simulink model "simulation_pipeline"  (R2023a)
settings: Solver=VariableStepAuto  StartTime=0.0  StopTime=10  FixedStep=1/2000  RelTol=1e-3
model workspace (MAT data in the model file):
  a = Simulink.Parameter
  a.Value = [0.16054 0.65442]
  a.DataType = 'auto'
  a.Complexity = 'real'
  a.Dimensions = [1 2]
  b = Simulink.Parameter
  b.Value = [0.16054 0.65442 1]
  b.DataType = 'auto'
  b.Complexity = 'real'
  b.Dimensions = [1 3]
  c = Simulink.Parameter
  c.Value = [1 1]
  c.DataType = 'auto'
  c.Complexity = 'real'
  c.Dimensions = [1 2]
  g = Simulink.Parameter
  g.Value = 0.00080298
  g.DataType = 'auto'
  g.Complexity = 'real'
  g.Dimensions = [1 1]
undefined symbols (not defined in the file): firhalfband
libraries: dspmlti4 x3, msbAdcFoundation x1, dspsigops x1, dspquant2 x1
settings Model: Creator=Lester  LastModifiedBy=Lester
settings DataIOCC: ReturnWorkspaceOutputs=off

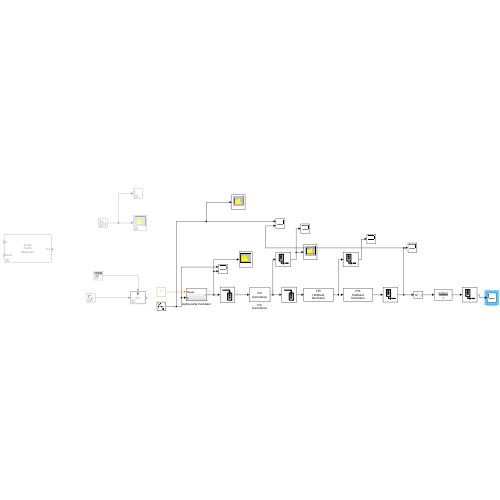
[thumbnail: Simulink's stored preview of the top-level diagram]
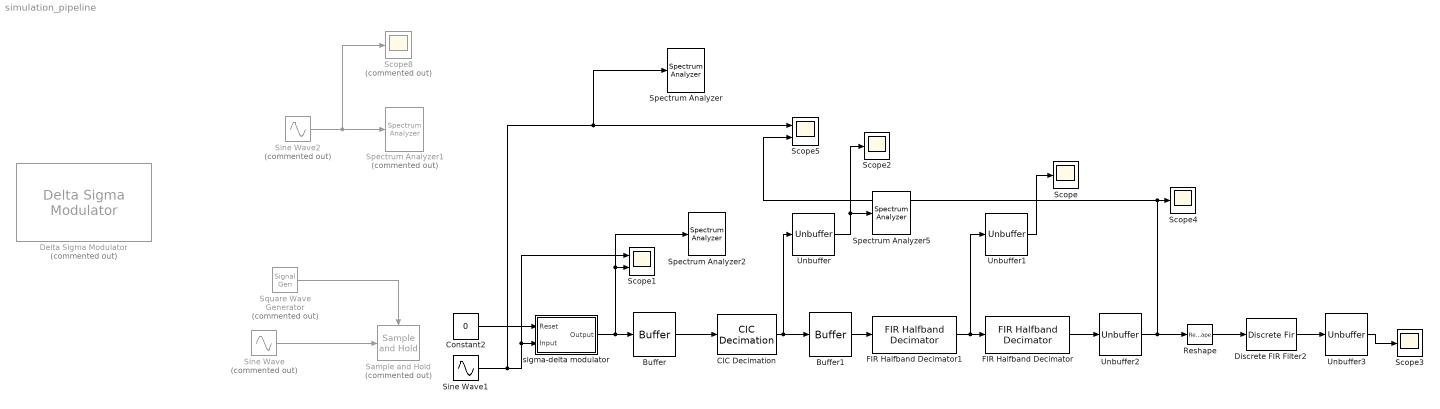
== system simulation_pipeline ==
  Buffer : Buffer  N=24  OutputFrames=off
  Buffer1 : Buffer  N=8  OutputFrames=off
  CIC Decimation : dspmlti4/CIC Decimation  filtFrom=Dialog parameters  filtobj=CICDECIM  ftype=Decimator  R=12  M=1  N=4  filterInternals=Full precision  BPS=[16 16 16 16]  FLPS=0  outputWordLength=32  outputFracLength=0  launchFVT=off  framing=Maintain input frame rate  RateOptions=Enforce single-rate processing
      settings: LibrarySourceBlock=|
      | dsphdlsupportfiltering/CIC
      | Decimation
  Constant2 : Constant  Value=0  SampleTime=1/2.304e6
  Delta Sigma Modulator : msbAdcFoundation/Delta Sigma Modulator  Commented=on  dsmArchitecture=CIFB  dsmOrder=2nd order  SamplingFrequency=128e3  NumberLevels=2  QuantizerOutput=[-1;1]  a=[0.1601 0.6515]  g=[0.0]  b=[0.1601 0.6515 1]  c=[1 1]  EnableNoise=on  SNR=75  InputPower=0.125  BandWidth=1000
      link override Delta Sigma Modulator: LabelModeActiveChoice=2CIFB
      link override Noise: LabelModeActiveChoice=noise
  Discrete FIR Filter2 : DiscreteFir  Coefficients=|  SampleTime=96e3
      | [-0.000958177958379201246547074433124180359
      | -0.003782484366489099070901547250400653866
      | -0.008055996906683227792855817028794263024
      | -0.010365278062492658955884294869065342937
      | -0.00550473485434811379835018385620060144 
      |  0.008631607068306285449055259562101127813
      |  0.025719525280152786411713705660986306611
      |  0.031614424562770325477512045608818880282
      |  0.014320649256157549564227871030652750051
      | -0.022003543765387822972456888237502425909
      | -0.051505493094117581198698729849638766609
      | -0.038973297856755691193075819001023774035
      |  0.034481095551837454005195127137994859368
      |  0.150902569099642724914644986711209639907
      |  0.25888391496113211109886265148816164583 
      |  0.302836379627961560512261485200724564493
      |  0.25888391496113211109886265148816164583 
      |  0.150902569099642724914644986711209639907
      |  0.034481095551837454005195127137994859368
      | -0.038973297856755691193075819001023774035
      | -0.051505493094117581198698729849638766609
      | -0.022003543765387822972456888237502425909
      |  0.014320649256157549564227871030652750051
      |  0.031614424562770325477512045608818880282
      |  0.025719525280152786411713705660986306611
      |  0.008631607068306285449055259562101127813
      | -0.00550473485434811379835018385620060144 
      | -0.010365278062492658955884294869065342937
      | -0.008055996906683227792855817028794263024
      | -0.003782484366489099070901547250400653866
      | -0.000958177958379201246547074433124180359]
  FIR Halfband Decimator : dspmlti4/FIR Halfband Decimator  Specification=Filter order and stopband attenuation  FilterOrder=14  TransitionWidth=4.1e3  StopbandAttenuation=100  DesignMethod=Auto  Numerator=firhalfband( 'minorder', 0.407, 1e-4 )  FilterBankOutputPort=off  InheritSampleRate=off  SampleRate=96e3  SimulateUsing=Code generation  roundingMode=Floor  coeffsDataTypeStr=fixdt(1,16)
  FIR Halfband Decimator1 : dspmlti4/FIR Halfband Decimator  Specification=Filter order and stopband attenuation  FilterOrder=14  TransitionWidth=4.1e3  StopbandAttenuation=100  DesignMethod=Auto  Numerator=firhalfband( 'minorder', 0.407, 1e-4 )  FilterBankOutputPort=off  InheritSampleRate=off  SampleRate=2*96e3  SimulateUsing=Code generation  roundingMode=Floor  coeffsDataTypeStr=fixdt(1,16)
  Reshape : Reshape  OutputDimensions=[1,2]
  Sample and Hold : dspsigops/Sample and Hold  Commented=on  trig=Rising edge  initCond=0  latchinput=off
  Scope{,2..4} (4 alike) : Scope
  Scope1 : Scope  NumInputPorts=2
  Scope5 : Scope  NumInputPorts=2
  Scope8 : Scope  Commented=on
  Sine Wave : Sin  Commented=on  Frequency=2*pi*100  SampleTime=1/2.304e6
  Sine Wave1 : Sin  Frequency=2*pi*100  SampleTime=1/2.304e6
  Sine Wave2 : Sin  Commented=on  Frequency=2*pi*100  SampleTime=1/2000
  Spectrum Analyzer : SpectrumAnalyzer  WindowPosition=[1.000000,49.000000,1707.000000,889.000000,]  ScopeFrameLocation=window  SpectrumType=Power density  SpectrumUnits=dBm/Hz  YLimits=[-308.65856886,26.07461712]  ColorLimits=[-80 20]
  Spectrum Analyzer1 : SpectrumAnalyzer  Commented=on  WindowPosition=[1.000000,49.000000,1707.000000,889.000000,]  ScopeFrameLocation=window  YLimits=[-240.74775427,-25.54872748]  ColorLimits=[-80 20]
  Spectrum Analyzer2 : SpectrumAnalyzer  WindowPosition=[1.000000,49.000000,1707.000000,889.000000,]  ScopeFrameLocation=window  SpectrumType=Power density  SpectrumUnits=dBm/Hz  YLimits=[-107.56343722,4.98269637]  ColorLimits=[-80 20]
  Spectrum Analyzer5 : SpectrumAnalyzer  WindowPosition=[1.000000,49.000000,1707.000000,889.000000,]  ScopeFrameLocation=window  SpectrumType=Power density  SpectrumUnits=dBm/Hz  YLimits=[-25.98451667,95.0310336]  ColorLimits=[-80 20]
  Square Wave Generator : SignalGenerator  Commented=on  WaveForm=square  Frequency=2.304e6  VectorParams1D=off
  Unbuffer{,1..3} (4 alike) : Unbuffer
  sigma-delta modulator : Subsystem
  wires:
  Square Wave Generator/1 -> Sample and Hold/Trigger
  Sine Wave/1 -> Sample and Hold/1
  Constant2/1 -> sigma-delta modulator/1(Reset)
  sigma-delta modulator/1(Output) -> Buffer/1, Spectrum Analyzer2/1, Scope1/2
  CIC Decimation/1 -> Unbuffer/1, Buffer1/1
  FIR Halfband Decimator1/1 -> Unbuffer1/1, FIR Halfband Decimator/1
  FIR Halfband Decimator/1 -> Unbuffer2/1
  Buffer/1 -> CIC Decimation/1
  Sine Wave1/1 -> Spectrum Analyzer/1, Scope5/1, Scope1/1, sigma-delta modulator/2(Input)
  Buffer1/1 -> FIR Halfband Decimator1/1
  Unbuffer/1 -> Spectrum Analyzer5/1, Scope2/1
  Unbuffer1/1 -> Scope/1
  Unbuffer2/1 -> Scope5/2, Scope4/1, Reshape/1
  Sine Wave2/1 -> Spectrum Analyzer1/1, Scope8/1
  Reshape/1 -> Discrete FIR Filter2/1
  Unbuffer3/1 -> Scope3/1
  Discrete FIR Filter2/1 -> Unbuffer3/1

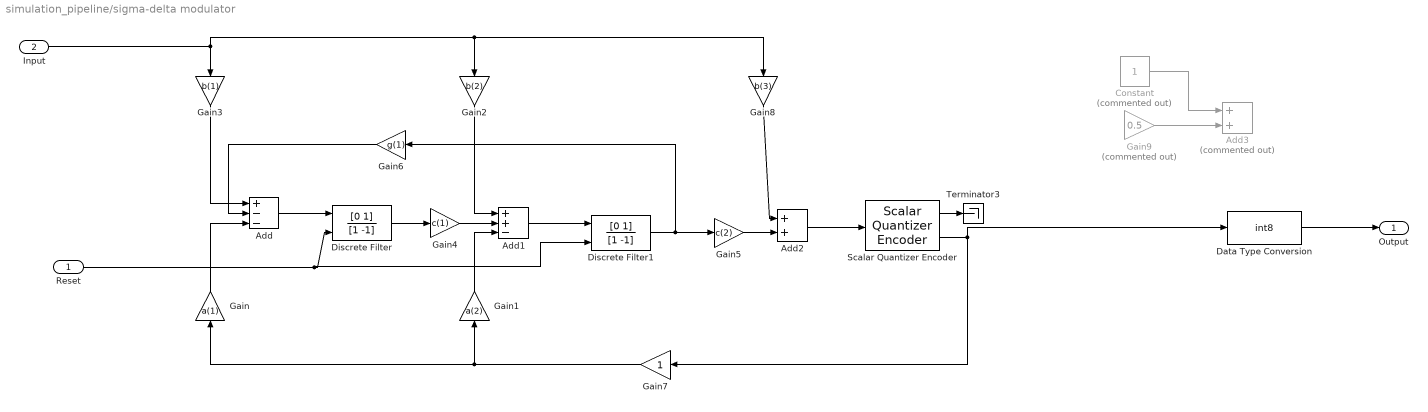
== system simulation_pipeline/sigma-delta modulator ==
  Reset : Inport
  Input : Inport  Port=2
  Add : Sum  Inputs=+--
  Add1 : Sum  Inputs=++-
  Add2 : Sum
  Add3 : Sum  Commented=on
  Constant : Constant  Commented=on
  Data Type Conversion : DataTypeConversion  OutDataTypeStr=int8  SaturateOnIntegerOverflow=off  RndMeth=Floor
  Discrete Filter : DiscreteFilter  Numerator=[0 1]  Denominator=[1 -1]  ExternalReset=Rising  SampleTime=1/2.304e6
      settings: InputPortMap=u0,r7
  Discrete Filter1 : DiscreteFilter  Numerator=[0 1]  Denominator=[1 -1]  ExternalReset=Rising  SampleTime=1/2.304e6
      settings: InputPortMap=u0,r7
  Gain : Gain  Gain=a(1)
  Gain1 : Gain  Gain=a(2)
  Gain2 : Gain  Gain=b(2)
  Gain3 : Gain  Gain=b(1)
  Gain4 : Gain  Gain=c(1)
  Gain5 : Gain  Gain=c(2)
  Gain6 : Gain  Gain=g(1)
  Gain7 : Gain
  Gain8 : Gain  Gain=b(3)
  Gain9 : Gain  Commented=on  Gain=0.5
  Scalar Quantizer Encoder : dspquant2/Scalar Quantizer Encoder  paramSrc=Specify via dialog  partType=Bounded  BBoundary=[-2/2:2/2]  UBoundary=[2:9]  SearchMethod=Linear  tieBreakRule=Choose the lower index  outQU=on  outQError=off  codebook=[-1, 1]  outStatus=off  invalidin=Clip  idtype=int8  roundingMode=Floor  overflowMode=off
  Terminator3 : Terminator
  Output : Outport
  wires:
  Gain5/1 -> Add2/2
  Input/1 -> Gain8/1, Gain2/1, Gain3/1
  Discrete Filter1/1 -> Gain5/1, Gain6/1
  Gain/1 -> Add/3
  Gain6/1 -> Add/2
  Gain2/1 -> Add1/1
  Add1/1 -> Discrete Filter1/1
  Gain4/1 -> Add1/2
  Discrete Filter/1 -> Gain4/1
  Gain3/1 -> Add/1
  Add2/1 -> Scalar Quantizer Encoder/1
  Gain8/1 -> Add2/1
  Reset/1 -> Discrete Filter/2, Discrete Filter1/2
  Gain7/1 -> Gain/1, Gain1/1
  Add/1 -> Discrete Filter/1
  Gain1/1 -> Add1/3
  Scalar Quantizer Encoder/1 -> Terminator3/1
  Scalar Quantizer Encoder/2 -> Data Type Conversion/1, Gain7/1
  Data Type Conversion/1 -> Output/1
  Gain9/1 -> Add3/2
  Constant/1 -> Add3/1
